simulink model "model"  (R2022a)
settings: Solver=ode45  StartTime=0.0  StopTime=1  MaxStep=1e-5  RelTol=1e-3
undefined symbols (not defined in the file or in its folder): plecs
libraries: simulink x1
settings Model: Creator=LIU  LastModifiedBy=LIU

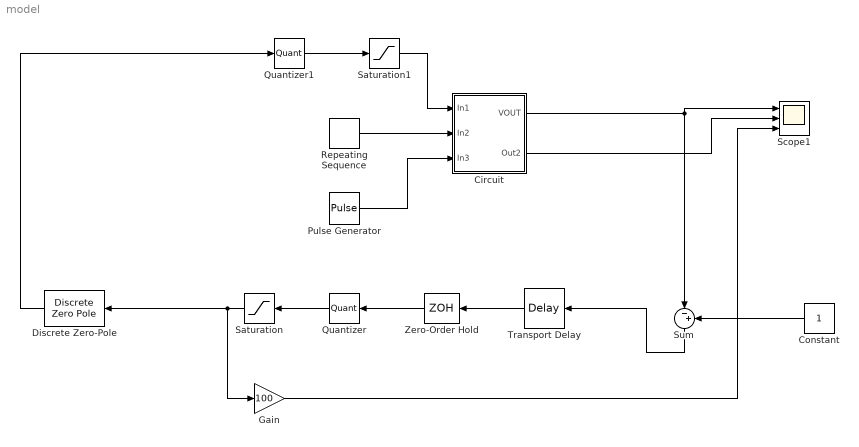
== system model ==
  Circuit : Subsystem  LoadFcn=plecs('sl', 200);  InitFcn=plecs('sl', 214);  StartFcn=plecs('sl', 208);  StopFcn=plecs('sl', 209);  mask(PlecsCircuit){PLECSData=<binary blob, 3272 chars, not shown>}
      mask prompts: PLECSData "PLECS Data (Do not delete or modify!)"
      mask init:
      | % PLACE CUSTOM INITIALIZATIONS ABOVE
      | % DO NOT REMOVE
      | plecs('sl', 215);
      | % DO NOT REMOVE
      settings: CopyFcn=plecs('sl', 203);  DeleteFcn=plecs('sl', 205);  UndoDeleteFcn=plecs('sl', 206);  PreSaveFcn=plecs('sl', 211);  PostSaveFcn=plecs('sl', 201);  NameChangeFcn=plecs('sl', 210);  DestroyFcn=plecs('sl', 207);  PreCopyFcn=plecs('sl', 216);  OpenFcn=plecs('sl', 202);  ErrorFcn=plerrorfcn
      mask Help: web(['file:///' fullfile(plecsdoc, 'creatingacircuit.html')])
      mask Display: disp('PLECS\nCircuit')
  Constant : Constant
  Discrete Zero-Pole : DiscreteZeroPole  Zeros=[0.9771 0.9425]  Poles=[1 -0.6367]  Gain=10.566  SampleTime=-1
  Gain : Gain  Gain=100
  Pulse Generator : DiscretePulseGenerator  PulseType=Time based  Period=0.1  PulseWidth=50
  Quantizer : Quantizer  QuantizationInterval=15.625e-3
  Quantizer1 : Quantizer  QuantizationInterval=1/256
  Repeating Sequence : simulink/Sources/Repeating Sequence  rep_seq_t=[0 2e-6]  rep_seq_y=[0 3]
  Saturation : Saturate  UpperLimit=62.5e-3  LowerLimit=-62.5e-3
  Saturation1 : Saturate  UpperLimit=0.95  LowerLimit=0.05
  Scope1 : Scope  NumInputPorts=3
  Sum : Sum  Inputs=|-+
  Transport Delay : TransportDelay  DelayTime=495e-9
  Zero-Order Hold : ZeroOrderHold  SampleTime=2e-6
  wires:
  Transport Delay/1 -> Zero-Order Hold/1
  Zero-Order Hold/1 -> Quantizer/1
  Quantizer/1 -> Saturation/1
  Quantizer1/1 -> Saturation1/1
  Circuit/1(VOUT) -> Sum/1, Scope1/1
  Circuit/2(Out2) -> Scope1/2
  Saturation1/1 -> Circuit/1(In1)
  Constant/1 -> Sum/2
  Sum/1 -> Transport Delay/1
  Saturation/1 -> Gain/1, Discrete Zero-Pole/1
  Discrete Zero-Pole/1 -> Quantizer1/1
  Gain/1 -> Scope1/3
  Repeating Sequence/1 -> Circuit/2(In2)
  Pulse Generator/1 -> Circuit/3(In3)

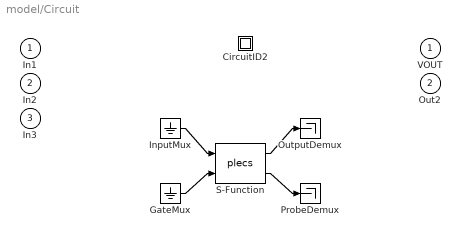
== system model/Circuit ==
  In1 : Inport  PortDimensions=1
  In2 : Inport  Port=2  PortDimensions=1
  In3 : Inport  Port=3  PortDimensions=1
  " CircuitID2 " : Subsystem
  " GateMux " : Ground
  " InputMux " : Ground
  " OutputDemux " : Terminator
  " ProbeDemux " : Terminator
  " S-Function " : S-Function  FunctionName=plecs  SFunctionDeploymentMode=off  EnableBusSupport=off
  VOUT : Outport  PortDimensions=1
  Out2 : Outport  Port=2  PortDimensions=1
  wires:
  " InputMux "/1 -> " S-Function "/1
  " GateMux "/1 -> " S-Function "/2
  " S-Function "/1 -> " OutputDemux "/1
  " S-Function "/2 -> " ProbeDemux "/1

== system model/Circuit/ CircuitID2  ==
